simulink model "lab04es02a_schema"  (R2021b)
settings: Solver=VariableStepAuto  StartTime=0.0  StopTime=10.0  RelTol=1e-3
values from neighbouring files (symbols this model uses):
  s = tf('s')    [L_04_05_21_es_stabilita_marginale.m]    (also in L_11_05_21_reti_anticipatrici.m; L_11_05_21_reti_anticipatrici_2.m; L_12_05_21_Esercizio_progetto_di_un_controllore.m; L_12_05_21_effetti_sul_comando.m)
libraries: cstblocks x3
settings Model: Creator=francescafornasier  LastModifiedBy=francescafornasier

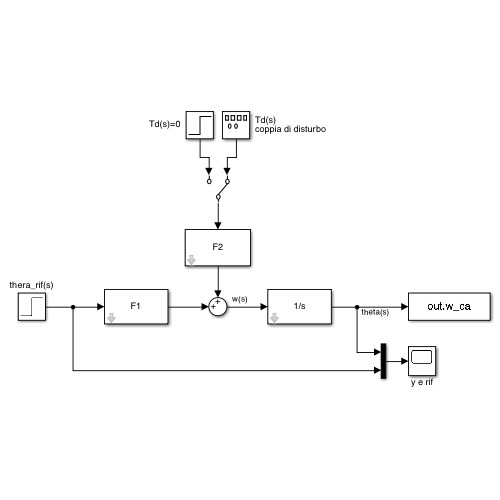
[thumbnail: Simulink's stored preview of the top-level diagram]
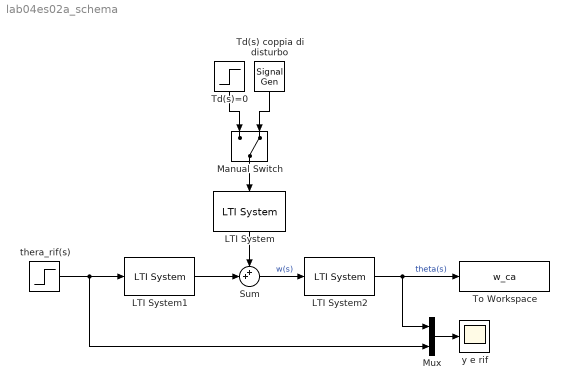
== system lab04es02a_schema ==
  LTI System : cstblocks/LTI System  sys=F2  IC=[]
  LTI System1 : cstblocks/LTI System  sys=F1  IC=[]
  LTI System2 : cstblocks/LTI System  sys=1/s  IC=[]
  Manual Switch : ManualSwitch  CurrentSetting=0
  Mux : Mux  Inputs=2
  Sum : Sum  Inputs=++|
  Td(s) coppia di disturbo : SignalGenerator  WaveForm=square  Amplitude=0.05  Frequency=0.1
  Td(s)=0 : Step  Time=0  After=0  SampleTime=0
  To Workspace : ToWorkspace  VariableName=w_ca  SaveFormat=Timeseries  SampleTime=-1
  thera_rif(s) : Step  Time=0  SampleTime=0
  y e rif : Scope
  wires:
  LTI System/1 -> Sum/1
  Td(s) coppia di disturbo/1 -> Manual Switch/2
  Td(s)=0/1 -> Manual Switch/1
  LTI System1/1 -> Sum/2
  Mux/1 -> y e rif/1
  Manual Switch/1 -> LTI System/1
  thera_rif(s)/1 -> Mux/2, LTI System1/1
  Sum/1 -> LTI System2/1  "w(s)"
  LTI System2/1 -> Mux/1, To Workspace/1  "theta(s)"
